simulink model "CLEARModelDetector"  (R2016b)
settings: Solver=FixedStepDiscrete  StartTime=0.0  StopTime=inf  FixedStep=sCoreParams.core.stepPeriod  RelTol=1e-3  EnableMultiTasking=on
undefined symbols (not defined in the file): neuralModelParams, sCoreParams
libraries: dspswit3 x2, simulink x1
settings Model: Creator=anish  LastModifiedBy=rzelmann
settings SolverCC: EnableConcurrentExecution=on  ConcurrentTasks=on
settings DataIOCC: SaveFormat=StructureWithTime  SignalLoggingSaveFormat=ModelDataLogs  SaveOutput=off  SignalLogging=off  DSMLogging=off  SaveTime=off
settings OptimizationCC: BlockReduction=off  ConditionallyExecuteInputs=off  DefaultParameterBehavior=Inlined  OptimizeBlockIOStorage=off  BufferReuse=off  GlobalBufferReuse=off  ExpressionFolding=off  LocalBlockOutputs=off  LifeSpan=inf
settings DebuggingCC: SignalRangeChecking=error  SaveWithParameterizedLinksMsg=none  AllowSymbolicDim=off  ModelReferenceSymbolNameMessage=none  StateNameClashWarn=warning  SFUnexpectedBacktrackingDiag=warning  SFNoUnconditionalDefaultTransitionDiag=warning  SFExecutionAtInitializationDiag=none
settings HardwareCC: ProdBitPerPointer=32  ProdBitPerSizeT=32  ProdBitPerPtrDiffT=32  ProdLargestAtomicFloat=None  ProdWordSize=32  ProdLongLongMode=on  ProdHWDeviceType=Generic->32-bit x86 compatible  TargetBitPerPointer=64  TargetLargestAtomicFloat=Float  TargetLongLongMode=on  TargetIntDivRoundTo=Zero  TargetEndianess=LittleEndian  TargetWordSize=64  TargetHWDeviceType=Intel->x86-64 (Windows64)
settings ModelReferenceCC: UpdateModelReferenceTargets=Force  ModelReferenceNumInstancesAllowed=Single  ModelReferencePassRootInputsByReference=off
settings RTWCC: SystemTargetFile=slrt.tlc  TemplateMakefile=slrt_default_tmf  Description=Simulink Real-Time  BuildConfiguration=Faster Runs  RTWCompilerOptimization=on
settings ConfigComp: CovMetricSettings=dw  CovHtmlReporting=on  CovSaveCumulativeToWorkspaceVar=on  CovSaveSingleToWorkspaceVar=on  CovExternalEMLEnable=off  CovSFcnEnable=off

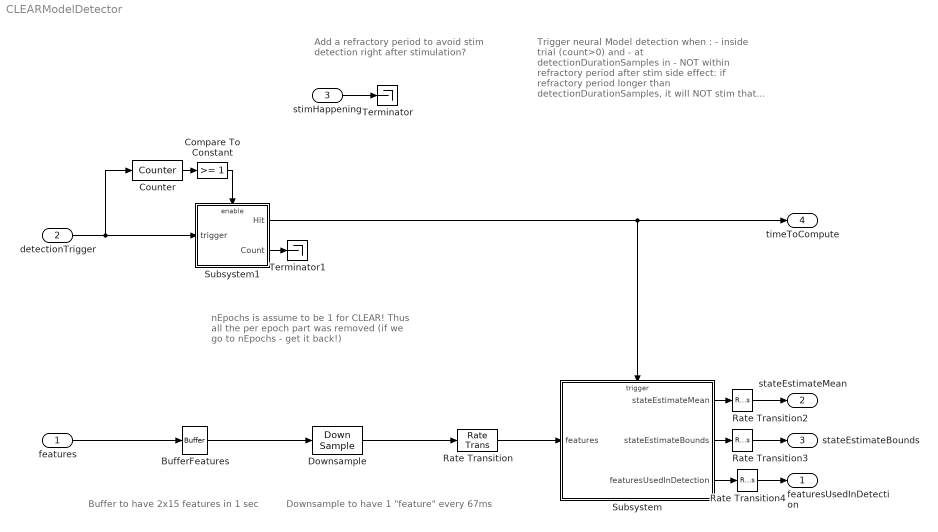
== system CLEARModelDetector ==
  note: Buffer to have 2x15 features in 1 sec
  note: Downsample to have 1 "feature" every 67ms
  note: nEpochs is assume to be 1 for CLEAR!
      | Thus all the per epoch part was removed
      |  (if we go to nEpochs - get it back!)
  note: Trigger neural Model detection when :
      |  -  inside trial (count>0) and
      | -  at detectionDurationSamples in
      | - NOT within refractory period after stim
      | side effect: if refractory period longer than detectionDurationSamples, it will NOT stim that next trial
  note: Add a refractory period to avoid
      | stim detection right after stimulation?
  features : Inport  PortDimensions=[1 neuralModelParams.nFeatures]
  detectionTrigger : Inport  Port=2  OutDataTypeStr=boolean  SampleTime=sCoreParams.core.stepPeriod
  stimHappening : Inport  Port=3  OutDataTypeStr=boolean  SampleTime=sCoreParams.core.stepPeriod
  BufferFeatures : Buffer  N=sCoreParams.decoders.txDetector.detectionDurationSteps  V=sCoreParams.decoders.txDetector.detectionDurationSteps - 1  TreatMby1Signals=One channel  OutputFrames=off
  Compare To Constant : simulink/Logic and Bit Operations/Compare To Constant  relop=>=  const=1  OutDataTypeStr=boolean
  Counter : dspswit3/Counter  Direction=Up  CountEvent=Rising edge  CounterSize=32 bits  MaxCount=sCoreParams.decoders.txDetector.detectionDurationSamples *5  InitialCount=0  Output=Count  HitValue=sCoreParams.decoders.txDetector.detectionDurationSamples  ResetInput=off  SamplesPerFrame=1  Ts=-1  CntDtype=double  HitDtype=Logical
  Downsample : DownSample  N=ceil(sCoreParams.decoders.txDetector.detectionDurationSteps/ neuralModelParams.nDataPoints)
  Rate Transition{,2..4} (4 alike) : RateTransition
  Subsystem : Subsystem
  Subsystem1 : Subsystem
  Terminator : Terminator
  Terminator1 : Terminator
  featuresUsedInDetection : Outport  PortDimensions=[neuralModelParams.nDataPoints neuralModelParams.nFeatures]
  stateEstimateMean : Outport  Port=2  PortDimensions=1
  stateEstimateBounds : Outport  Port=3  PortDimensions=[1 2]
  timeToCompute : Outport  Port=4  PortDimensions=1
  wires:
  Subsystem/1(stateEstimateMean) -> Rate Transition2/1
  stimHappening/1 -> Terminator/1
  detectionTrigger/1 -> Subsystem1/1(trigger), Counter/1
  Subsystem/3(featuresUsedInDetection) -> Rate Transition4/1
  Subsystem/2(stateEstimateBounds) -> Rate Transition3/1
  Subsystem1/1(Hit) -> timeToCompute/1, Subsystem/Trigger
  Compare To Constant/1 -> Subsystem1/Enable
  Counter/1 -> Compare To Constant/1
  Rate Transition/1 -> Subsystem/1(features)
  Rate Transition2/1 -> stateEstimateMean/1
  Rate Transition3/1 -> stateEstimateBounds/1
  Rate Transition4/1 -> featuresUsedInDetection/1
  Subsystem1/2(Count) -> Terminator1/1
  Downsample/1 -> Rate Transition/1
  BufferFeatures/1 -> Downsample/1
  features/1 -> BufferFeatures/1

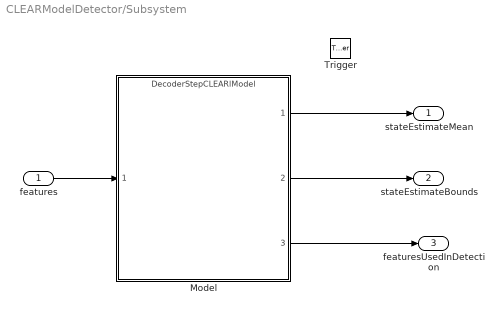
== system CLEARModelDetector/Subsystem ==
  features : Inport
  Trigger : TriggerPort  VariantControl=Variant  PortDimensions=1
  Model : ModelReference  ModelNameDialog=DecoderStepCLEARlModel.slx  SimulationMode=Normal  ModelReferenceVersion=1.504
  stateEstimateMean : Outport  InitialOutput=-500
  stateEstimateBounds : Outport  Port=2  InitialOutput=[-500 -500]
  featuresUsedInDetection : Outport  Port=3
  wires:
  features/1 -> Model/1
  Model/3 -> featuresUsedInDetection/1
  Model/2 -> stateEstimateBounds/1
  Model/1 -> stateEstimateMean/1

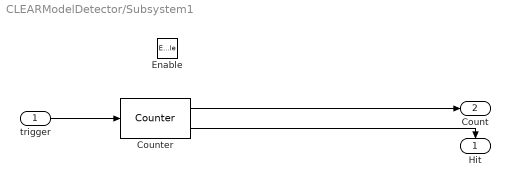
== system CLEARModelDetector/Subsystem1 ==
  trigger : Inport
  Enable : EnablePort
  Counter : dspswit3/Counter  Direction=Up  CountEvent=Free running  CounterSize=32 bits  MaxCount=sCoreParams.decoders.txDetector.detectionDurationSamples *5  InitialCount=1  Output=Count and Hit  HitValue=ceil(sCoreParams.decoders.txDetector.detectionDurationSteps)  ResetInput=on  SamplesPerFrame=1  Ts=-1  CntDtype=double  HitDtype=Logical
  Hit : Outport
  Count : Outport  Port=2  InitialOutput=1
  wires:
  Counter/1 -> Count/1
  Counter/2 -> Hit/1
  trigger/1 -> Counter/1
